simulink model "optical_flow_webcam"  (R2012b)
settings: Solver=ode45  StartTime=0.0  StopTime=10.0  RelTol=1e-3
undefined symbols (not defined in the file): gray, Horn, magnitude, none, Rec, Schunck, SDTV, strel, videoinput
libraries: visionsinks x4, visionanalysis x2, visionstatistics x2, visionconversions x1, visiontextngfix x1, imaqlib x1, visionmorphops x1
settings Model: Creator=dagoodma  LastModifiedBy=dagoodma

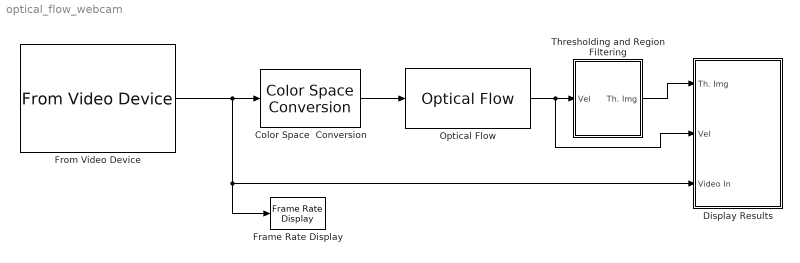
== system optical_flow_webcam ==
  Color Space  Conversion : visionconversions/Color Space  Conversion  conversion=Obsolete  conversionActive=R'G'B' to intensity  wp_str=D65  rec=Rec. 601 (SDTV)  sys=1125/60/2:1  imagePorts=One multidimensional signal
  Display Results : Subsystem
  Frame Rate Display : visionsinks/Frame Rate Display  UpdateRate=10
  From Video Device : imaqlib/From Video Device  DeviceMenu=macvideo 1 (Built-in iSight)  Device=macvideo 1 (Built-in iSight)  ObjConstructor=videoinput('macvideo', 1)  VideoFormatMenu=YCbCr422_640x480  VideoFormat=YCbCr422_640x480  VideoSource=default  ROIPosition=[0 0 480 640]  EnableHWTrigger=off  TriggerConfiguration=none/none  SampleTime=1/30  OutputPortsMode=One multidimensional signal  DataType=single  CanDoHWTrigger=no  ReturnedColorSpace=rgb  BlockHandle=2027.0005  ROIWidth=640  ROIHeight=480  ROIColumn=0  ROIRow=0  EngXMLPath=/Applications/MATLAB_R2012b.app/toolbox/imaq/imaq/private  DevXMLPath=/Applications/MATLAB_R2012b.app/toolbox/imaq/imaqadaptors/maci64  EngLibPath=/Applications/MATLAB_R2012b.app/toolbox/imaq/imaqblks/imaqmex/maci64  ColorSpace=rgb  BayerSensorAlignment=grbg
  Optical Flow : visionanalysis/Optical Flow  method=Horn-Schunck  gradMethod=Difference filter [-1 1]  which2img=Current frame and N-th frame back  N=1  outVelForm=Horizontal and vertical components in complex form  lambda=1  stop_criteria=When maximum number of iterations is reached  maxAllowAbsDiff=eps  maxIter=10  numInports=3  sigmaS=1.5  sigmaW=1  eigTh=0.0039  discardNormalFlow=off  outputCurrentImage=off  prodOutputMode=Binary point scaling  prodOutputWordLength=32  prodOutputFracLength=20  outputMode=Binary point scaling  outputWordLength=32  outputFracLength=20  roundingMode=Nearest  overflowMode=on
  Thresholding and Region Filtering : Subsystem
  wires:
  From Video Device/1 -> Color Space  Conversion/1, Display Results/3(Video In), Frame Rate Display/1
  Color Space  Conversion/1 -> Optical Flow/1
  Optical Flow/1 -> Display Results/2(Vel), Thresholding and Region Filtering/1(Vel)
  Thresholding and Region Filtering/1(Th. Img) -> Display Results/1(Th. Img)

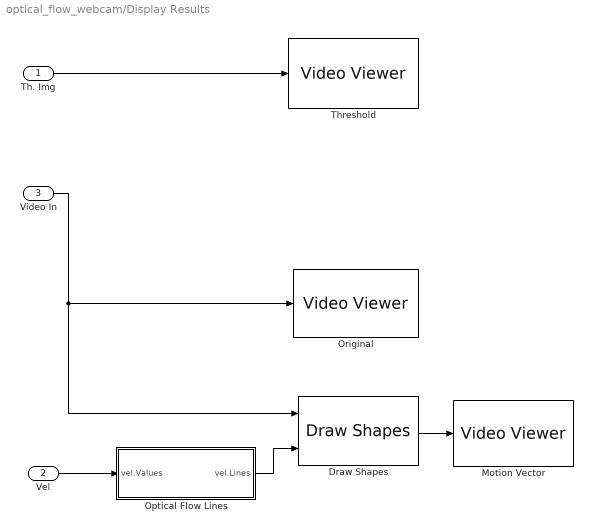
== system optical_flow_webcam/Display Results ==
  Th. Img : Inport
  Vel : Inport  Port=2
  Video In : Inport  Port=3
  Draw Shapes : visiontextngfix/Draw Shapes  shape=Lines  fill=off  fillClrSource=Specify via dialog  display=User-specified value  intensity=200  color=[255 255 0]  opacity=0.6  viewport=Entire image  antialiasing=off  inType=Obsolete  imagePorts=One multidimensional signal  prodOutputMode=Binary point scaling  prodOutputWordLength=32  prodOutputFracLength=14  memoryMode=Specify word length  memoryWordLength=16  memoryFracLength=15  roundingMode=Floor  overflowMode=off
  Motion Vector : visionsinks/Video Viewer  inputType=Obsolete7b  imagePorts=One multidimensional signal  useColorMap=off  colormapValue=gray(256)  specRange=off  minInputVal=0  maxInputVal=255  FigPos=[311 564 313 366]  AxisZoom=on  trueSizedOnce=on  OpenAtMdlStart=on  DefaultConfigurationName=vipscopes.VideoViewerScopeCfg
  Optical Flow Lines : Subsystem  mask(Optical Flow Lines){scaleFactor=20}
      mask prompts: scaleFactor "Motion vector gain:"
      mask help: Generates the coordinate points of optical flow lines.
      mask Help: Generates the coordinate points of optical flow lines. Look under its mask to see the implementation details.
  Original : visionsinks/Video Viewer  inputType=Obsolete7b  imagePorts=One multidimensional signal  useColorMap=off  colormapValue=gray(256)  specRange=off  minInputVal=0  maxInputVal=255  FigPos=[-4 588 344 347]  AxisZoom=on  trueSizedOnce=on  OpenAtMdlStart=on  DefaultConfigurationName=vipscopes.VideoViewerScopeCfg
  Threshold : visionsinks/Video Viewer  inputType=Obsolete7b  imagePorts=One multidimensional signal  useColorMap=off  colormapValue=gray(256)  specRange=off  minInputVal=0  maxInputVal=255  FigPos=[702 571 447 370]  AxisZoom=on  trueSizedOnce=on  OpenAtMdlStart=on  DefaultConfigurationName=vipscopes.VideoViewerScopeCfg
  wires:
  Video In/1 -> Original/1, Draw Shapes/1
  Th. Img/1 -> Threshold/1
  Draw Shapes/1 -> Motion Vector/1
  Optical Flow Lines/1(vel.Lines) -> Draw Shapes/2
  Vel/1 -> Optical Flow Lines/1(vel.Values)

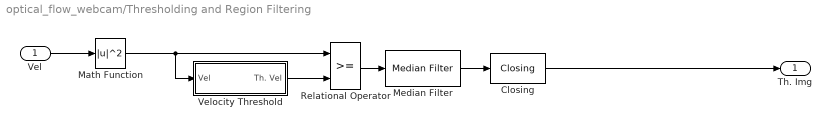
== system optical_flow_webcam/Thresholding and Region Filtering ==
  Vel : Inport
  Closing : visionmorphops/Closing  nhoodsrc=Specify via dialog  strel=strel('line',6,45)
  Math Function : Math  Operator=magnitude^2  SaturateOnIntegerOverflow=on
  Median Filter : visionanalysis/Median Filter  nghbood=[3 3]  outSize=Same as input port I  padType=Constant  padSrc=Specify via dialog  padVal=1  roundingMode=Floor  overflowMode=off
  Relational Operator : RelationalOperator  OutDataTypeStr=boolean
  Velocity Threshold : Subsystem
  Th. Img : Outport
  wires:
  Closing/1 -> Th. Img/1
  Median Filter/1 -> Closing/1
  Velocity Threshold/1(Th. Vel) -> Relational Operator/2
  Vel/1 -> Math Function/1
  Relational Operator/1 -> Median Filter/1
  Math Function/1 -> Velocity Threshold/1(Vel), Relational Operator/1

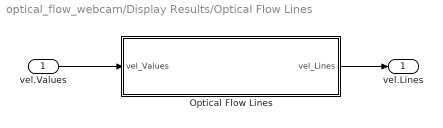
== system optical_flow_webcam/Display Results/Optical Flow Lines ==
  vel.Values : Inport
  Optical Flow Lines : MATLAB Function  TreatAsAtomicUnit=on
  vel.Lines : Outport
  wires:
  Optical Flow Lines/1(vel_Lines) -> vel.Lines/1
  vel.Values/1 -> Optical Flow Lines/1(vel_Values)

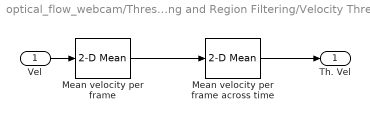
== system optical_flow_webcam/Thresholding and Region Filtering/Velocity Threshold ==
  Vel : Inport
  Mean velocity per frame : visionstatistics/2-D Mean  run=off  reset_popup=None  directionMode=Entire input  dimension=1  treatSBRowAsCol=on  roiEnable=off  roiType=Rectangles  roiPortion=Entire ROI  roiOutput=Individual statistics for each ROI  roiFlag=off  outputDataTypeStr=Inherit: Same as accumulator  outputLastDataTypeStr=Inherit: Same as accumulator  outputMin=[]  outputMax=[]  accumMode=Binary point scaling  accumWordLength=32  accumFracLength=0  accumDataTypeStr=fixdt([],32,0)  accumLastDataTypeStr=fixdt([],32,0)  roundingMode=Floor  overflowMode=off
  Mean velocity per frame across time : visionstatistics/2-D Mean  run=on  reset_popup=None  directionMode=Entire input  dimension=1  treatSBRowAsCol=on  roiEnable=off  roiType=Rectangles  roiPortion=Entire ROI  roiOutput=Individual statistics for each ROI  roiFlag=off  outputDataTypeStr=Inherit: Same as accumulator  outputLastDataTypeStr=Inherit: Same as accumulator  outputMin=[]  outputMax=[]  accumMode=Binary point scaling  accumWordLength=32  accumFracLength=0  accumDataTypeStr=fixdt([],32,0)  accumLastDataTypeStr=fixdt([],32,0)  roundingMode=Floor  overflowMode=off
  Th. Vel : Outport
  wires:
  Mean velocity per frame across time/1 -> Th. Vel/1
  Vel/1 -> Mean velocity per frame/1
  Mean velocity per frame/1 -> Mean velocity per frame across time/1

== matlab function optical_flow_webcam/Display Results/Optical Flow Lines/Optical Flow Lines ==
  data: vel_Values input; vel_Lines output; scaleFactor parameter size=1
function vel_Lines=OpticalFlowLines(vel_Values, scaleFactor) 

% Generates the coordinate points of optical flow lines

persistent first_time;
persistent X;
persistent Y;
persistent RV;
persistent CV;
if isempty(first_time)
    first_time     = 1;
    %% user may change the following three parameters
    borderOffset   = 5;
    decimFactorRow = 5;
    decimFactorCol = 5;    
    %%
    [R C] = size(vel_Values);
    RV = borderOffset:decimFactorRow:(R-borderOffset);   
    CV = borderOffset:decimFactorCol:(C-borderOffset);
    [Y X] = meshgrid(CV,RV);
end

tmp = vel_Values(RV,CV);
tmp = tmp.*scaleFactor;
vel_Lines = [Y(:), X(:), Y(:)+real(tmp(:)), X(:)+imag(tmp(:))];
